simulink library "BOBLibrary"  (R2019b)
settings: Solver=VariableStepAuto  StartTime=0.0  StopTime=10.0  RelTol=1e-3
libraries: arduinolib x3
settings Model: Creator=matej  LastModifiedBy=matej

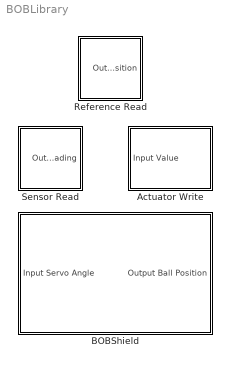
== system BOBLibrary ==
  Actuator Write : Subsystem  mask{InputType=Percentage (%), RangeType=Default values (recommended), MinAngle=-30, MaxAngle=30, Ts=0.025}
      mask prompts: InputType "Input type"; RangeType "Angle range"; MinAngle "Minimal angle  (°)"; MaxAngle "Maximal angle  (°)"; Ts "Sampling period (s)"
      mask init:
      | if InputType==1 
      | MinInput = 0;
      | MaxInput = 100;
      | elseif InputType==2
      | MinInput = 5;
      | MaxInput = 100;            
      | end
      mask TypeOptions InputType: Percentage (%) | Distance (mm)
      mask TypeOptions RangeType: Default values (recommended) | Manual values
      mask Callback RangeType:
      | CurrentBlock = gcb;
      | Type = get_param(CurrentBlock,'RangeType');
      | Menu = Simulink.Mask.get(CurrentBlock);
      | Min = Menu.getParameter('MinAngle');
      | Max = Menu.getParameter('MaxAngle');
      | 
      | if strcmp(Type,'Default values (recommended)')
      | Min.Enabled='off';
      | Max.Enabled='off';
      | elseif strcmp(Type,'Manual values')
      | Min.Enabled='on';
      | Max.Enabled='on';
      | end
      mask DialogControl DescGroupVar Prompt: BOBShield Servo Drive
      mask DialogControl DescTextVar Prompt: Maps input value and then sets the servo drive angle in choosen range
      mask DialogControl Inputs Prompt: Inputs
      mask DialogControl MinAngle Tooltip: Recommended -30
      mask DialogControl MaxAngle Tooltip: Recommended +30
      mask Display: image('assets\BOBFig\Servo.svg');
  BOBShield : Subsystem  mask{OutType=Percentage (%), Ncal=100, Ts=0.025}
      mask prompts: OutType "Output type"; Ncal "Calibration samples (-)"; Ts "Sampling period (s):"
      mask TypeOptions OutType: Percentage (%) | Position (mm)
      mask DialogControl DescGroupVar Prompt: BOBShield
      mask DialogControl DescTextVar Prompt: The block represents a BOBShield device. It accepts an input signal in the range of 0-100% which controls the angle of the servo drive and outputs the position of the ball in the form selected by the user. The block performs the calibration at the beginning of the simulation and therefore requires a sampling period and number of calibration samples out of which the extreme reading values will be computed using their mean value.
      mask Display: image('assets\BOBFig\BOB1.svg');
  Reference Read : Subsystem  mask{ReadoutRadio=Analog value (ADC), Ts=0.025}
      mask prompts: ReadoutRadio "Readout type"; Ts "Sampling period (s):"
      mask init:
      | if ReadoutRadio==1 
      | GainVal = (100/1023);                               
      | elseif ReadoutRadio==2
      | GainVal = (5/1023);                     
      | else
      | GainVal = 1;             
      | end
      mask TypeOptions ReadoutRadio: Percentage (%) | Voltage (V) | Analog value (ADC)
      mask DialogControl DescGroupVar Prompt: BOBShield Potentiometer
      mask DialogControl DescTextVar Prompt: The block represents potentiometer runner on the BOBShield device. User can choose the form of block output that represents the current potentiometer runner position.
      mask Display: image('assets\Potentiometer.svg');
  Sensor Read : Subsystem  mask{OutRadio=Distance (mm), CalType=Manual values, MinVal=5, MaxVal=100, Ts=0.025}
      mask prompts: OutRadio "Output type"; CalType "Calibration values:"; MinVal "Minimal reading (mm):"; MaxVal "Maximal reading (mm):"; Ts "Sampling period (s):"
      mask init:
      | if CalType==1    
      |     set_param(gcb,'MinVal',num2str(5));
      |     set_param(gcb,'MaxVal',num2str(100));    
      | end
      mask TypeOptions OutRadio: Distance (mm) | Position (mm) | Percentage (%)
      mask Callback OutRadio:
      | CurrentBlock = gcb;
      | Output = get_param(CurrentBlock,'OutRadio');
      | Calib = get_param(CurrentBlock,'CalType');
      | Menu = Simulink.Mask.get(CurrentBlock);
      | CalibOpt = Menu.getParameter('CalType');
      | MinOpt = Menu.getParameter('MinVal');
      | MaxOpt = Menu.getParameter('MaxVal');
      | 
      | if strcmp(Output,'Distance (mm)')
      | CalibOpt.Enabled='off';
      | MinOpt.Enabled='off';
      | MaxOpt.Enabled='off';
      | elseif strcmp(Calib,'Manual values')
      | CalibOpt.Enabled='on';
      | MinOpt.Enabled='on';
      | MaxOpt.Enabled='on';
      | else
      | CalibOpt.Enabled='on';
      | MinOpt.Enabled='off';
      | MaxOpt.Enabled='off';
      | end
      mask TypeOptions CalType: Default values (recommended) | Manual values
      mask Callback CalType:
      | CurrentBlock = gcbh;
      | Output = get_param(CurrentBlock,'OutRadio');
      | Calib = get_param(CurrentBlock,'CalType');
      | Menu = Simulink.Mask.get(CurrentBlock);
      | MinOpt = Menu.getParameter('MinVal');
      | MaxOpt = Menu.getParameter('MaxVal');
      | 
      | if strcmp(Output,'Distance (mm)')
      | MinOpt.Enabled='off';
      | MaxOpt.Enabled='off';
      | elseif strcmp(Calib,'Manual values')
      | MinOpt.Enabled='on';
      | MaxOpt.Enabled='on';
      | else
      | MinOpt.Enabled='off';
      | MaxOpt.Enabled='off';
      | end
      mask DialogControl DescGroupVar Prompt: BOBShield Distance Sensor
      mask DialogControl DescTextVar Prompt: The block represents the I2C Time of Flight VL6180x Distance Sensor on the BOBShield device. User can choose type of reading this block outputs. For Percentage output, calibration values are required. By default the most probable values are used, but if needed they can be manually set. User can also specify sampling period in seconds.
      mask DialogControl MinVal Tooltip: Recommended 5 mm.
      mask DialogControl MaxVal Tooltip: Recommended 100 mm.
      mask Display: image('assets\TOF.svg');

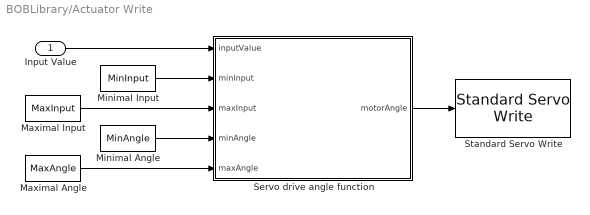
== system BOBLibrary/Actuator Write ==
  Input Value : Inport  SampleTime=Ts
  Maximal Angle : Constant  Value=MaxAngle  SampleTime=Ts
  Maximal Input : Constant  Value=MaxInput  SampleTime=Ts
  Minimal Angle : Constant  Value=MinAngle  SampleTime=Ts
  Minimal Input : Constant  Value=MinInput  SampleTime=Ts
  Servo drive angle function : MATLAB Function  TreatAsAtomicUnit=on
  Standard Servo Write : arduinolib/Standard Servo Write  pinNumber=9  ServoIndex=0  blockPlatform=ARDUINO
      settings: SourceProductName=Simulink Support Package for Arduino Hardware
  wires:
  Input Value/1 -> Servo drive angle function/1(inputValue)
  Minimal Angle/1 -> Servo drive angle function/4(minAngle)
  Minimal Input/1 -> Servo drive angle function/2(minInput)
  Maximal Input/1 -> Servo drive angle function/3(maxInput)
  Maximal Angle/1 -> Servo drive angle function/5(maxAngle)
  Servo drive angle function/1(motorAngle) -> Standard Servo Write/1

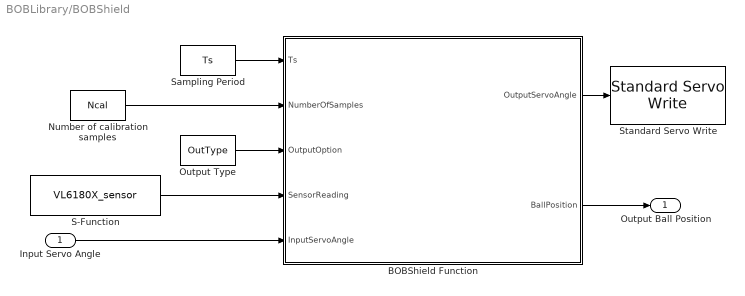
== system BOBLibrary/BOBShield ==
  Input Servo Angle : Inport
  BOBShield Function : MATLAB Function  TreatAsAtomicUnit=on
  Number of calibration samples : Constant  Value=Ncal  SampleTime=Ts
  Output Type : Constant  Value=OutType  SampleTime=Ts
  S-Function : S-Function  FunctionName=VL6180X_sensor  SFunctionModules='VL6180X_sensor_wrapper'  SFunctionDeploymentMode=off  EnableBusSupport=off
  Sampling Period : Constant  Value=Ts  SampleTime=Ts
  Standard Servo Write : arduinolib/Standard Servo Write  pinNumber=9  ServoIndex=0  blockPlatform=ARDUINO
      settings: SourceProductName=Simulink Support Package for Arduino Hardware
  Output Ball Position : Outport  VectorParamsAs1DForOutWhenUnconnected=off
  wires:
  BOBShield Function/2(BallPosition) -> Output Ball Position/1
  S-Function/1 -> BOBShield Function/4(SensorReading)
  Input Servo Angle/1 -> BOBShield Function/5(InputServoAngle)
  Sampling Period/1 -> BOBShield Function/1(Ts)
  Output Type/1 -> BOBShield Function/3(OutputOption)
  BOBShield Function/1(OutputServoAngle) -> Standard Servo Write/1
  Number of calibration samples/1 -> BOBShield Function/2(NumberOfSamples)

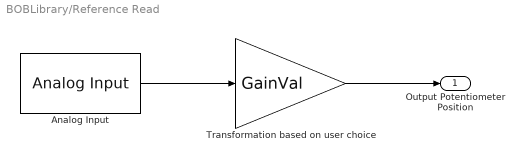
== system BOBLibrary/Reference Read ==
  Analog Input : arduinolib/Analog Input  pinNumber=0  ReadResultsOnly=off  ConversionTriggerSource=Software  ExternalTriggerType=uint32(0)  OutputDataType=uint16  EnableConversionCompleteNotify=off  EnableOuputStatus=off  SampleTime=Ts  blockPlatform=arduino
  Transformation based on user choice : Gain  Gain=GainVal  ParamDataTypeStr=double
  "Output Potentiometer Position " : Outport  VectorParamsAs1DForOutWhenUnconnected=off
  wires:
  Transformation based on user choice/1 -> "Output Potentiometer Position "/1
  Analog Input/1 -> Transformation based on user choice/1

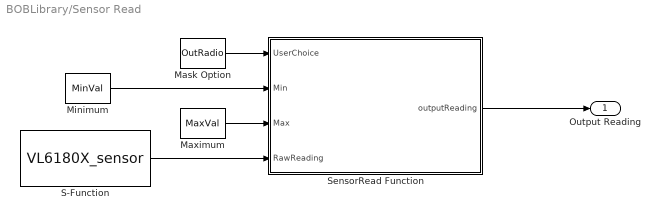
== system BOBLibrary/Sensor Read ==
  Mask Option : Constant  Value=OutRadio  SampleTime=Ts
  Maximum : Constant  Value=MaxVal  SampleTime=Ts
  Minimum : Constant  Value=MinVal  SampleTime=Ts
  S-Function : S-Function  FunctionName=VL6180X_sensor  SFunctionModules='VL6180X_sensor_wrapper'  SFunctionDeploymentMode=off  EnableBusSupport=off
  SensorRead Function : MATLAB Function  TreatAsAtomicUnit=on
  Output Reading : Outport  SampleTime=Ts  VectorParamsAs1DForOutWhenUnconnected=off
  wires:
  Mask Option/1 -> SensorRead Function/1(UserChoice)
  S-Function/1 -> SensorRead Function/4(RawReading)
  Maximum/1 -> SensorRead Function/3(Max)
  Minimum/1 -> SensorRead Function/2(Min)
  SensorRead Function/1(outputReading) -> Output Reading/1

== matlab function BOBLibrary/Sensor Read/SensorRead Function ==
  data: UserChoice input; outputReading output; Min input; Max input; RawReading input
%     Matlab function for Sensor Read block functionality.
%
%     This code is part of the AutomationShield hardware and software
%     ecosystem. Visit http://www.automationshield.com for more
%     details. This code is licensed under a Creative Commons
%     Attribution-NonCommercial 4.0 International License.
%
%     Created by Matej Simovec
%     Last update: 27.12.2020.

function outputReading = fcn(UserChoice, Min, Max, RawReading)

if UserChoice == 1
    outputReading = constrain(RawReading, 10, 100);
elseif UserChoice == 2
    outputReading = constrain(map(RawReading, Max, Min, 0, Max-Min), 0, Max);
else
    outputReading = constrain(map(RawReading, Max, Min, 0, 100), 0, 100);
end

end

== matlab function BOBLibrary/BOBShield/BOBShield Function ==
  data: Ts input; NumberOfSamples input; OutputOption input; SensorReading input; InputServoAngle input; OutputServoAngle output; BallPosition output
%     Matlab function for BOBShield block functionality.
%
%     This code is part of the AutomationShield hardware and software
%     ecosystem. Visit http://www.automationshield.com for more
%     details. This code is licensed under a Creative Commons
%     Attribution-NonCommercial 4.0 International License.
%
%     Edited by Matej Šimovec
%     Last update: 28.12.2020.

function [OutputServoAngle, BallPosition] = fcn(Ts, NumberOfSamples, OutputOption, SensorReading, InputServoAngle)

persistent calibrationStatus iteration time minVal maxVal; % Persistent variables

if isempty(iteration)                                      % Initialisation
    iteration = 0;
    time = 0;
    calibrationStatus = 0;
    minVal = 0;
    maxVal = 0;
end  

SensorReading = constrain(SensorReading, 10, 80);   % Avoid invalid readings

if calibrationStatus == 0                                    % Getting minimal value
    OutputServoAngle = 60;                                  % Set power output to max
    BallPosition = 0;
    if SensorReading > 70                              % Wait for ball to go to the opposite side of the sensor
        time = time + Ts;
        if time >= 1                                       % Wait 1 second to stabilise
            iteration = iteration + 1;
            minVal = minVal + SensorReading;
            if iteration == NumberOfSamples
                minVal = minVal / NumberOfSamples;         % As average of N samples
                calibrationStatus = 1;
                time = 0;
                iteration = 0;
            end
        end
    end
elseif calibrationStatus == 1                              % Getting maximal value
    OutputServoAngle = 120;                                    % Set power output to zero
    BallPosition = 0;
    if SensorReading <= 20                             % Wait for ball to go to the sensor side
        time = time + Ts;
        if time >= 1                                       % Wait 1 second to stabilise
            iteration = iteration + 1;
            maxVal = maxVal + SensorReading;
            if iteration == NumberOfSamples
                maxVal = maxVal / NumberOfSamples;         % As average of N samples
                calibrationStatus = 2;
                time = 0;
                iteration = 0;
            end
        end
    end
else
    OutputServoAngle = constrain(InputServoAngle,60,120);
    if OutputOption == 1                                    % Output based on user choice
        %BallPosition = constrain(map(SensorReading, maxVal, minVal, 0, 100), 0, 100); %test
        BallPosition = constrain(map(SensorReading, minVal, maxVal, 0, 100), 0, 100);
    else
        BallPosition = constrain(map(SensorReading, maxVal, minVal, 0, maxVal-minVal), 0, maxVal);
    end
end

end

== matlab function BOBLibrary/Actuator Write/Servo drive angle function ==
  data: inputValue input; motorAngle output; minInput input; maxInput input; minAngle input; maxAngle input
function motorAngle = fcn(inputValue, minInput, maxInput, minAngle, maxAngle)

minAngle = 90 + minAngle;
maxAngle = 90 + maxAngle;

motorAngle = mapfun(inputValue,minInput,maxInput,minAngle, maxAngle);

end
